simulink model "unlinear"  (R2016b)
settings: Solver=VariableStepAuto  StartTime=0.0  StopTime=par.t12  RelTol=1e-3
values from neighbouring files (symbols this model uses):
  as = rmfield(as,'data')    [PrepareForModel (2).m]    (also in PrepareForModel.m)
  trj = rmfield(trj,'aerodata')    [ImportFromMatAndExcel.m]
undefined symbols (not defined in the file or in its folder): dm
libraries: aerolibschedule x4, simulink_extras x2
settings Model: Creator=ivan_  LastModifiedBy=ivan_

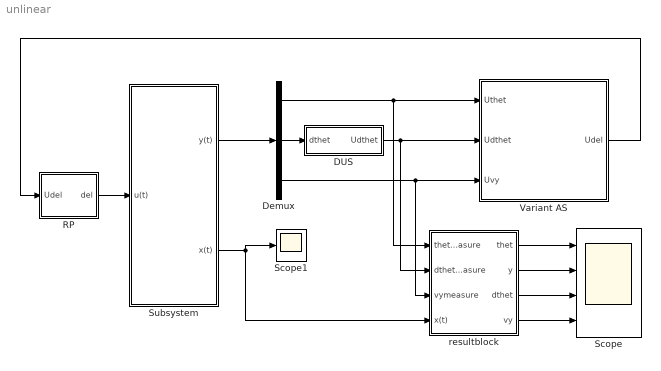
== system unlinear ==
  "DUS " : Subsystem
  Demux : Demux  Outputs=3
  RP : Subsystem
  Scope : Scope  NumInputPorts=4
  Scope1 : Scope
  Subsystem : Subsystem
  Variant AS : Subsystem  Variant=on  OverrideUsingVariant=Variant2
  resultblock : Subsystem
  wires:
  Demux/2 -> "DUS "/1(dthet)
  Variant AS/1(Udel) -> RP/1(Udel)
  Demux/1 -> resultblock/1(thetmeasure), Variant AS/1(Uthet)
  "DUS "/1(Udthet) -> resultblock/2(dthetmeasure), Variant AS/2(Udthet)
  Demux/3 -> resultblock/3(vymeasure), Variant AS/3(Uvy)
  RP/1(del) -> Subsystem/1(u(t))
  Subsystem/1(y(t)) -> Demux/1
  resultblock/1(thet) -> Scope/1
  resultblock/2(y) -> Scope/2
  resultblock/3(dthet) -> Scope/3
  resultblock/4(vy) -> Scope/4
  Subsystem/2(x(t)) -> Scope1/1, resultblock/4(x(t))

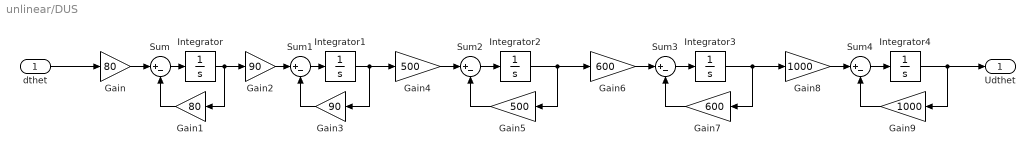
== system unlinear/DUS  ==
  dthet : Inport
  Gain : Gain  Gain=80
  Gain1 : Gain  Gain=80
  Gain2 : Gain  Gain=90
  Gain3 : Gain  Gain=90
  Gain4 : Gain  Gain=500
  Gain5 : Gain  Gain=500
  Gain6 : Gain  Gain=600
  Gain7 : Gain  Gain=600
  Gain8 : Gain  Gain=1000
  Gain9 : Gain  Gain=1000
  Integrator{,1..4} (5 alike) : Integrator
  Sum{,1..4} (5 alike) : Sum  Inputs=|+-
  Udthet : Outport
  wires:
  Sum/1 -> Integrator/1
  dthet/1 -> Gain/1
  Sum4/1 -> Integrator4/1
  Gain3/1 -> Sum1/2
  Integrator3/1 -> Gain8/1, Gain7/1
  Sum1/1 -> Integrator1/1
  Sum3/1 -> Integrator3/1
  Sum2/1 -> Integrator2/1
  Integrator4/1 -> Udthet/1, Gain9/1
  Gain5/1 -> Sum2/2
  Integrator2/1 -> Gain6/1, Gain5/1
  Integrator1/1 -> Gain4/1, Gain3/1
  Gain/1 -> Sum/1
  Gain4/1 -> Sum2/1
  Gain2/1 -> Sum1/1
  Gain8/1 -> Sum4/1
  Integrator/1 -> Gain2/1, Gain1/1
  Gain6/1 -> Sum3/1
  Gain1/1 -> Sum/2
  Gain7/1 -> Sum3/2
  Gain9/1 -> Sum4/2

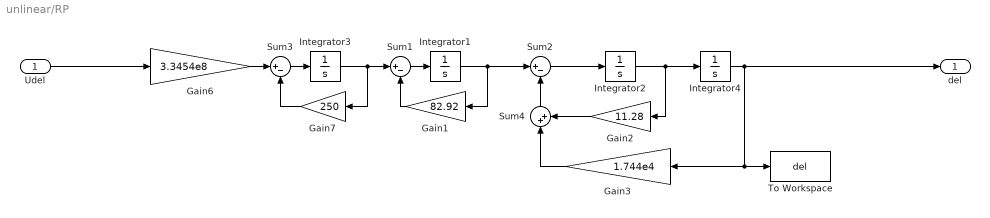
== system unlinear/RP ==
  Udel : Inport
  Gain1 : Gain  Gain=82.92
  Gain2 : Gain  Gain=11.28
  Gain3 : Gain  Gain=1.744e4
  Gain6 : Gain  Gain=3.3454e8
  Gain7 : Gain  Gain=250
  Integrator{1..4} (4 alike) : Integrator
  Sum1 : Sum  Inputs=|+-
  Sum2 : Sum  Inputs=|+-
  Sum3 : Sum  Inputs=|+-
  Sum4 : Sum  Inputs=|++
  To Workspace : ToWorkspace  VariableName=del  SaveFormat=Structure With Time  SampleTime=-1
      settings: StopFcn=|
      | res.del.val = del.signals.values;
      | res.del.t = del.time;
      | clear del;
  del : Outport
  wires:
  Udel/1 -> Gain6/1
  Integrator3/1 -> Sum1/1, Gain7/1
  Sum3/1 -> Integrator3/1
  Gain6/1 -> Sum3/1
  Integrator4/1 -> del/1, Gain3/1, To Workspace/1
  Sum4/1 -> Sum2/2
  Sum2/1 -> Integrator2/1
  Gain3/1 -> Sum4/1
  Gain2/1 -> Sum4/2
  Sum1/1 -> Integrator1/1
  Integrator2/1 -> Integrator4/1, Gain2/1
  Gain7/1 -> Sum3/2
  Integrator1/1 -> Sum2/1, Gain1/1
  Gain1/1 -> Sum1/2

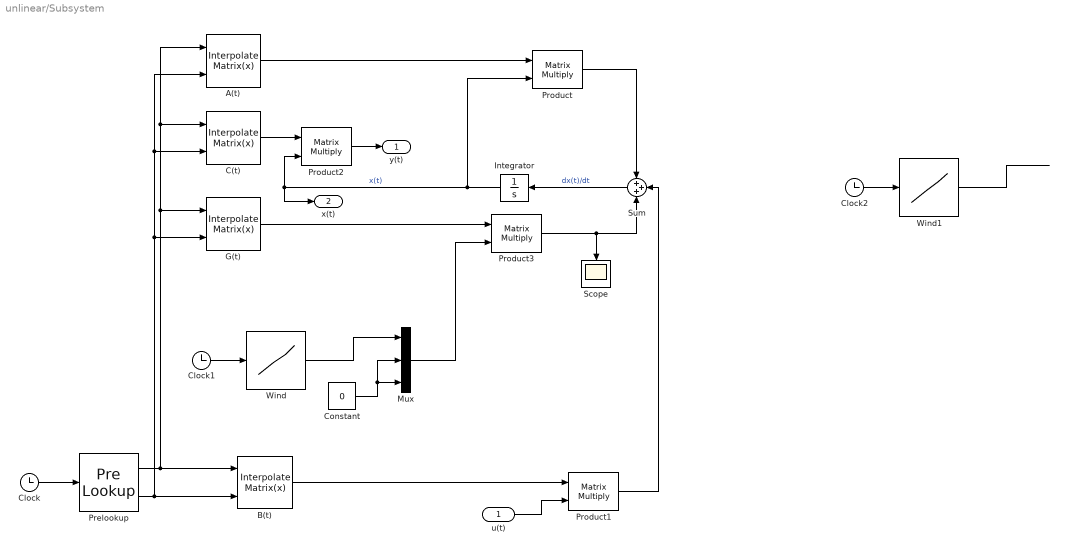
== system unlinear/Subsystem ==
  u(t) : Inport
  "A(t) " : aerolibschedule/Interpolate Matrix(x)   matrix=dm.A
  B(t) : aerolibschedule/Interpolate Matrix(x)   matrix=dm.B
  C(t) : aerolibschedule/Interpolate Matrix(x)   matrix=dm.C
  Clock : Clock
  Clock1 : Clock
  Clock2 : Clock
  Constant : Constant  Value=0
  G(t) : aerolibschedule/Interpolate Matrix(x)   matrix=dm.G
  Integrator : Integrator
  Mux : Mux  Inputs=3
  Prelookup : PreLookup  BreakpointsData=dm.t
  Product{,1..3} (4 alike) : Product  Multiplication=Matrix(*)
  Scope : Scope
  Sum : Sum  Inputs=+++
  Wind : Lookup_n-D  NumberOfTableDimensions=1  BreakpointsForDimension1=dm.t  Table=trj.wind  ExtrapMethod=Clip  UseLastTableValue=on  InternalRulePriority=Speed  RndMeth=Simplest  InputSameDT=on
  Wind1 : Lookup_n-D  NumberOfTableDimensions=1  BreakpointsForDimension1=dm.t  Table=trj.wind  ExtrapMethod=Clip  UseLastTableValue=on  InternalRulePriority=Speed  RndMeth=Simplest  InputSameDT=on
  y(t) : Outport
  x(t) : Outport  Port=2
  wires:
  Sum/1 -> Integrator/1  "dx(t)/dt"
  u(t)/1 -> Product1/2
  Integrator/1 -> Product/2, Product2/2, x(t)/1  "x(t)"
  Product2/1 -> y(t)/1
  Mux/1 -> Product3/2
  Product3/1 -> Sum/3, Scope/1
  G(t)/1 -> Product3/1
  "A(t) "/1 -> Product/1
  B(t)/1 -> Product1/1
  C(t)/1 -> Product2/1
  Wind/1 -> Mux/1
  Prelookup/2 -> "A(t) "/2, C(t)/2, G(t)/2, B(t)/2
  Prelookup/1 -> "A(t) "/1, C(t)/1, G(t)/1, B(t)/1
  Clock/1 -> Prelookup/1
  Product/1 -> Sum/1
  Clock1/1 -> Wind/1
  Product1/1 -> Sum/2
  Constant/1 -> Mux/3, Mux/2
  Wind1/1 -> ?
  Clock2/1 -> Wind1/1

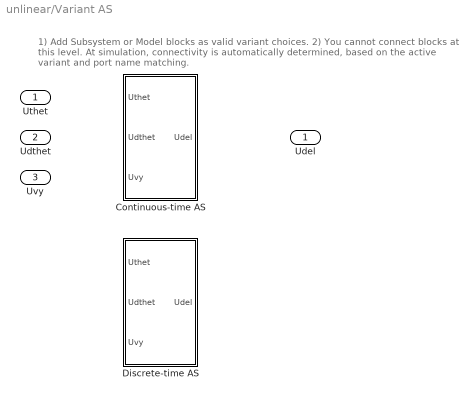
== system unlinear/Variant AS ==
  note: 1) Add Subsystem or Model blocks as valid variant choices.
      | 2) You cannot connect blocks at this level. At simulation, connectivity is automatically
      | determined, based on the active variant and port name matching.
  Uthet : Inport
  Udthet : Inport  Port=2
  Uvy : Inport  Port=3
  Continuous-time AS : Subsystem  VariantControl=Variant1
  Discrete-time AS : Subsystem  VariantControl=Variant2
  Udel : Outport

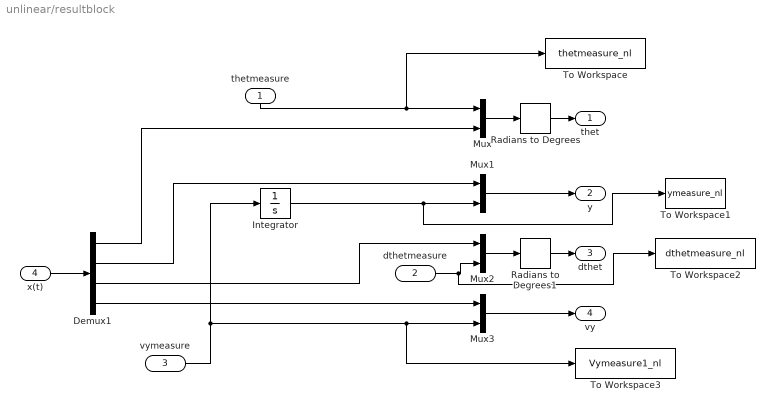
== system unlinear/resultblock ==
  thetmeasure : Inport
  dthetmeasure : Inport  Port=2
  vymeasure : Inport  Port=3
  x(t) : Inport  Port=4
  Demux1 : Demux
  Integrator : Integrator
  Mux{,1..3} (4 alike) : Mux  Inputs=2
  Radians to Degrees : simulink_extras/Transformations/Radians to Degrees
  Radians to Degrees1 : simulink_extras/Transformations/Radians to Degrees
  To Workspace : ToWorkspace  VariableName=thetmeasure_nl  SaveFormat=Structure With Time  SampleTime=-1
  To Workspace1 : ToWorkspace  VariableName=ymeasure_nl  SaveFormat=Structure With Time  SampleTime=-1
  To Workspace2 : ToWorkspace  VariableName=dthetmeasure_nl  SaveFormat=Structure With Time  SampleTime=-1
  To Workspace3 : ToWorkspace  VariableName=Vymeasure1_nl  SaveFormat=Structure With Time  SampleTime=-1
  thet : Outport
  y : Outport  Port=2
  dthet : Outport  Port=3
  vy : Outport  Port=4
  wires:
  x(t)/1 -> Demux1/1
  thetmeasure/1 -> To Workspace/1, Mux/1
  Integrator/1 -> To Workspace1/1, Mux1/2
  dthetmeasure/1 -> To Workspace2/1, Mux2/2
  Demux1/2 -> Mux1/1
  Demux1/3 -> Mux2/1
  Mux/1 -> Radians to Degrees/1
  Demux1/1 -> Mux/2
  Mux3/1 -> vy/1
  Demux1/4 -> Mux3/1
  vymeasure/1 -> Integrator/1, To Workspace3/1, Mux3/2
  Mux1/1 -> y/1
  Mux2/1 -> Radians to Degrees1/1
  Radians to Degrees1/1 -> dthet/1
  Radians to Degrees/1 -> thet/1

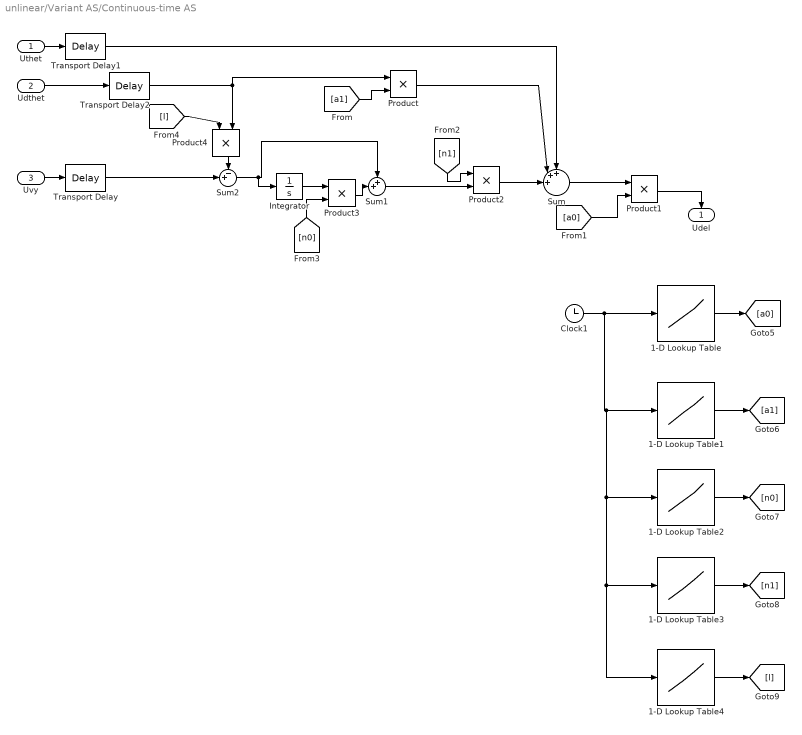
== system unlinear/Variant AS/Continuous-time AS ==
  Uthet : Inport
  Udthet : Inport  Port=2
  Uvy : Inport  Port=3
  1-D Lookup Table : Lookup_n-D  NumberOfTableDimensions=1  BreakpointsForDimension1=as.t  Table=as.a0  ExtrapMethod=Clip  UseLastTableValue=on  InternalRulePriority=Speed  RndMeth=Simplest  InputSameDT=on
  1-D Lookup Table1 : Lookup_n-D  NumberOfTableDimensions=1  BreakpointsForDimension1=as.t  Table=as.a1  ExtrapMethod=Clip  UseLastTableValue=on  InternalRulePriority=Speed  RndMeth=Simplest  InputSameDT=on
  1-D Lookup Table2 : Lookup_n-D  NumberOfTableDimensions=1  BreakpointsForDimension1=as.t  Table=as.n0  ExtrapMethod=Clip  UseLastTableValue=on  InternalRulePriority=Speed  RndMeth=Simplest  InputSameDT=on
  1-D Lookup Table3 : Lookup_n-D  NumberOfTableDimensions=1  BreakpointsForDimension1=as.t  Table=as.n1  ExtrapMethod=Clip  UseLastTableValue=on  InternalRulePriority=Speed  RndMeth=Simplest  InputSameDT=on
  1-D Lookup Table4 : Lookup_n-D  NumberOfTableDimensions=1  BreakpointsForDimension1=as.t  Table=as.l  ExtrapMethod=Clip  UseLastTableValue=on  InternalRulePriority=Speed  RndMeth=Simplest  InputSameDT=on
  Clock1 : Clock
  Integrator : Integrator
  Product{,1..4} (5 alike) : Product
  Sum : Sum  Inputs=+++||
  Sum1 : Sum  Inputs=++|
  Sum2 : Sum  Inputs=-+|
  Transport Delay : TransportDelay  DelayTime=[0.0214]
  Transport Delay1 : TransportDelay  DelayTime=[0.0214]
  Transport Delay2 : TransportDelay  DelayTime=[0.0114]
  Udel : Outport
  wires:
  Sum2/1 -> Integrator/1, Sum1/1
  Sum1/1 -> Product2/2
  Udthet/1 -> Transport Delay2/1
  Sum/1 -> Product1/1
  Product4/1 -> Sum2/1
  Product/1 -> Sum/2
  Uvy/1 -> Transport Delay/1
  Uthet/1 -> Transport Delay1/1
  [a1] -> Product/2
  [a0] -> Product1/2
  Product2/1 -> Sum/3
  Product1/1 -> Udel/1
  [l] -> Product4/1
  [n1] -> Product2/1
  1-D Lookup Table/1 -> [a0]
  1-D Lookup Table1/1 -> [a1]
  1-D Lookup Table2/1 -> [n0]
  1-D Lookup Table3/1 -> [n1]
  1-D Lookup Table4/1 -> [l]
  Clock1/1 -> 1-D Lookup Table4/1, 1-D Lookup Table3/1, 1-D Lookup Table2/1, 1-D Lookup Table1/1, 1-D Lookup Table/1
  [n0] -> Product3/2
  Integrator/1 -> Product3/1
  Product3/1 -> Sum1/2
  Transport Delay/1 -> Sum2/2
  Transport Delay1/1 -> Sum/1
  Transport Delay2/1 -> Product4/2, Product/1

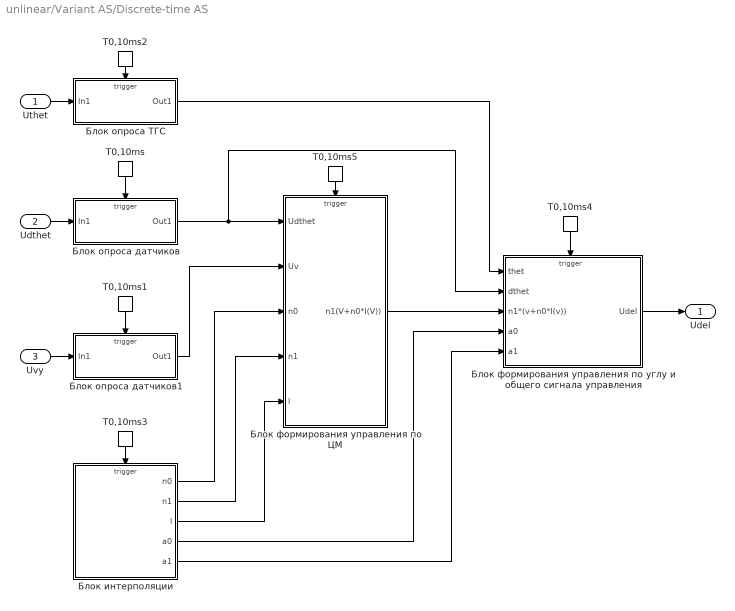
== system unlinear/Variant AS/Discrete-time AS ==
  Uthet : Inport
  Udthet : Inport  Port=2
  Uvy : Inport  Port=3
  T0,10ms : DiscretePulseGenerator  PulseType=Time based  Period=dm.T0  PulseWidth=10  PhaseDelay=0.012
  T0,10ms1 : DiscretePulseGenerator  PulseType=Time based  Period=dm.T0  PulseWidth=10
  T0,10ms2 : DiscretePulseGenerator  PulseType=Time based  Period=dm.T0  PulseWidth=10
  T0,10ms3 : DiscretePulseGenerator  PulseType=Time based  Period=dm.T0*4  PulseWidth=10  PhaseDelay=0.015
  T0,10ms4 : DiscretePulseGenerator  PulseType=Time based  Period=dm.T0  PulseWidth=10  PhaseDelay=0.021
  T0,10ms5 : DiscretePulseGenerator  PulseType=Time based  Period=dm.T0  PulseWidth=10  PhaseDelay=0.018
  Блок интерполяции : Subsystem
  Блок опроса ТГС : Subsystem  TreatAsAtomicUnit=on
  Блок опроса датчиков : Subsystem  TreatAsAtomicUnit=on
  Блок опроса датчиков1 : Subsystem  TreatAsAtomicUnit=on
  Блок формирования управления по углу и общего сигнала управления : Subsystem
  Блок формирования управления по ЦМ : Subsystem
  Udel : Outport
  wires:
  T0,10ms/1 -> Блок опроса датчиков/Trigger
  Udthet/1 -> Блок опроса датчиков/1(In1)
  T0,10ms1/1 -> Блок опроса датчиков1/Trigger
  Uvy/1 -> Блок опроса датчиков1/1(In1)
  T0,10ms2/1 -> Блок опроса ТГС/Trigger
  Uthet/1 -> Блок опроса ТГС/1(In1)
  Блок опроса датчиков/1(Out1) -> Блок формирования управления по углу и общего сигнала управления/2(dthet), Блок формирования управления по ЦМ/1(Udthet)
  Блок опроса датчиков1/1(Out1) -> Блок формирования управления по ЦМ/2(Uv)
  Блок опроса ТГС/1(Out1) -> Блок формирования управления по углу и общего сигнала управления/1(thet)
  Блок формирования управления по ЦМ/1(n1(V+n0*I(V))) -> Блок формирования управления по углу и общего сигнала управления/3(n1*(v+n0*I(v)))
  Блок формирования управления по углу и общего сигнала управления/1(Udel) -> Udel/1
  Блок интерполяции/4(a0) -> Блок формирования управления по углу и общего сигнала управления/4(a0)
  Блок интерполяции/5(a1) -> Блок формирования управления по углу и общего сигнала управления/5(a1)
  Блок интерполяции/2(n1) -> Блок формирования управления по ЦМ/4(n1)
  Блок интерполяции/3("l ") -> Блок формирования управления по ЦМ/5(l)
  Блок интерполяции/1(n0) -> Блок формирования управления по ЦМ/3(n0)
  T0,10ms3/1 -> Блок интерполяции/Trigger
  T0,10ms4/1 -> Блок формирования управления по углу и общего сигнала управления/Trigger
  T0,10ms5/1 -> Блок формирования управления по ЦМ/Trigger

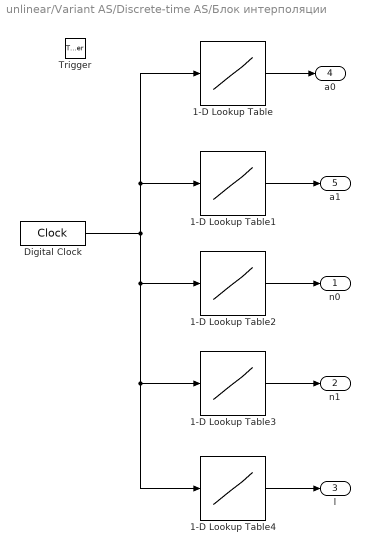
== system unlinear/Variant AS/Discrete-time AS/Блок интерполяции ==
  Trigger : TriggerPort  VariantControl=Variant
  1-D Lookup Table : Lookup_n-D  NumberOfTableDimensions=1  BreakpointsForDimension1=as.t  Table=as.a0  ExtrapMethod=Clip  UseLastTableValue=on  InternalRulePriority=Speed  RndMeth=Simplest  InputSameDT=on
  1-D Lookup Table1 : Lookup_n-D  NumberOfTableDimensions=1  BreakpointsForDimension1=as.t  Table=as.a1  ExtrapMethod=Clip  UseLastTableValue=on  InternalRulePriority=Speed  RndMeth=Simplest  InputSameDT=on
  1-D Lookup Table2 : Lookup_n-D  NumberOfTableDimensions=1  BreakpointsForDimension1=as.t  Table=as.n0  ExtrapMethod=Clip  UseLastTableValue=on  InternalRulePriority=Speed  RndMeth=Simplest  InputSameDT=on
  1-D Lookup Table3 : Lookup_n-D  NumberOfTableDimensions=1  BreakpointsForDimension1=as.t  Table=as.n1  ExtrapMethod=Clip  UseLastTableValue=on  InternalRulePriority=Speed  RndMeth=Simplest  InputSameDT=on
  1-D Lookup Table4 : Lookup_n-D  NumberOfTableDimensions=1  BreakpointsForDimension1=as.t  Table=as.l  ExtrapMethod=Clip  UseLastTableValue=on  InternalRulePriority=Speed  RndMeth=Simplest  InputSameDT=on
  Digital Clock : DigitalClock  SampleTime=-1
  n0 : Outport
  n1 : Outport  Port=2
  "l " : Outport  Port=3
  a0 : Outport  Port=4
  a1 : Outport  Port=5
  wires:
  1-D Lookup Table3/1 -> n1/1
  1-D Lookup Table2/1 -> n0/1
  1-D Lookup Table1/1 -> a1/1
  1-D Lookup Table/1 -> a0/1
  1-D Lookup Table4/1 -> "l "/1
  Digital Clock/1 -> 1-D Lookup Table/1, 1-D Lookup Table1/1, 1-D Lookup Table2/1, 1-D Lookup Table3/1, 1-D Lookup Table4/1

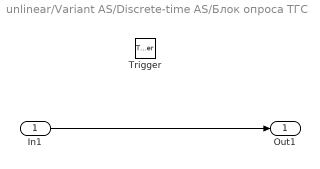
== system unlinear/Variant AS/Discrete-time AS/Блок опроса ТГС ==
  In1 : Inport
  Trigger : TriggerPort  VariantControl=Variant
  Out1 : Outport
  wires:
  In1/1 -> Out1/1

== system unlinear/Variant AS/Discrete-time AS/Блок опроса датчиков ==
  In1 : Inport
  Trigger : TriggerPort  VariantControl=Variant
  Out1 : Outport
  wires:
  In1/1 -> Out1/1

== system unlinear/Variant AS/Discrete-time AS/Блок опроса датчиков1 ==
  In1 : Inport
  Trigger : TriggerPort  VariantControl=Variant
  Out1 : Outport
  wires:
  In1/1 -> Out1/1

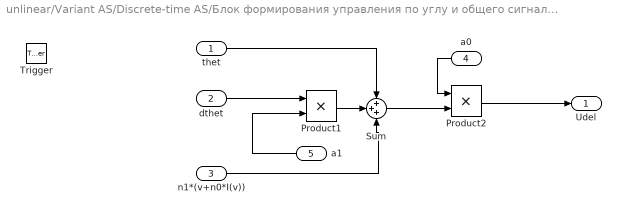
== system unlinear/Variant AS/Discrete-time AS/Блок формирования управления по углу и общего сигнала управления ==
  thet : Inport
  dthet : Inport  Port=2
  n1*(v+n0*I(v)) : Inport  Port=3
  a0 : Inport  Port=4
  a1 : Inport  Port=5
  Trigger : TriggerPort  VariantControl=Variant
  Product1 : Product
  Product2 : Product
  Sum : Sum  Inputs=+++
  Udel : Outport
  wires:
  Product1/1 -> Sum/2
  a0/1 -> Product2/1
  thet/1 -> Sum/1
  dthet/1 -> Product1/1
  n1*(v+n0*I(v))/1 -> Sum/3
  a1/1 -> Product1/2
  Product2/1 -> Udel/1
  Sum/1 -> Product2/2

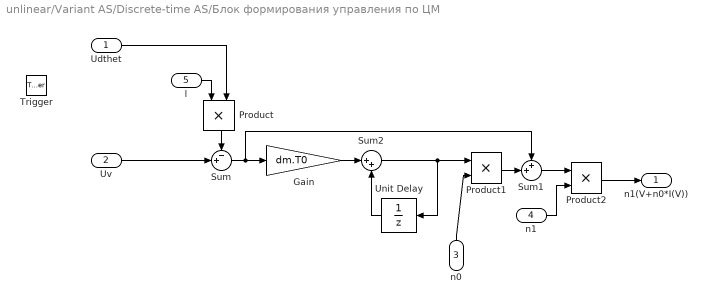
== system unlinear/Variant AS/Discrete-time AS/Блок формирования управления по ЦМ ==
  Udthet : Inport
  Uv : Inport  Port=2
  n0 : Inport  Port=3
  n1 : Inport  Port=4
  l : Inport  Port=5
  Trigger : TriggerPort  VariantControl=Variant
  Gain : Gain  Gain=dm.T0
  Product : Product
  Product1 : Product
  Product2 : Product
  Sum : Sum  Inputs=-+|
  Sum1 : Sum  Inputs=++|
  Sum2 : Sum  Inputs=|++
  Unit Delay : UnitDelay  SampleTime=-1
  n1(V+n0*I(V)) : Outport
  wires:
  Uv/1 -> Sum/2
  Sum1/1 -> Product2/1
  l/1 -> Product/1
  Udthet/1 -> Product/2
  Product/1 -> Sum/1
  Sum/1 -> Gain/1, Sum1/1
  n1/1 -> Product2/2
  Unit Delay/1 -> Sum2/2
  Product2/1 -> n1(V+n0*I(V))/1
  Gain/1 -> Sum2/1
  Sum2/1 -> Product1/1, Unit Delay/1
  n0/1 -> Product1/2
  Product1/1 -> Sum1/2
